simulink model "model2"  (R2022b)
settings: Solver=VariableStepAuto  StartTime=0.0  StopTime=0.5  RelTol=1e-3
libraries: simulink x1
settings Model: Creator=NINGMEI  LastModifiedBy=NINGMEI

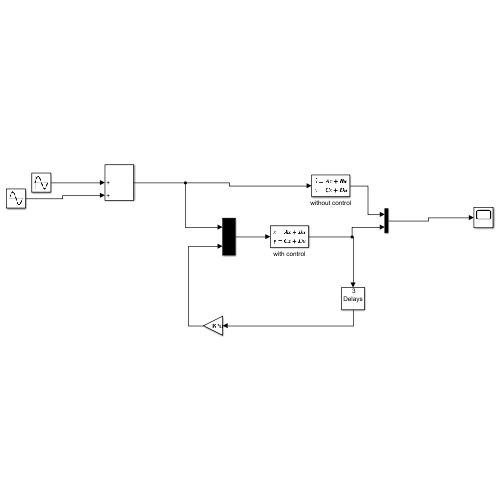
[thumbnail: Simulink's stored preview of the top-level diagram]
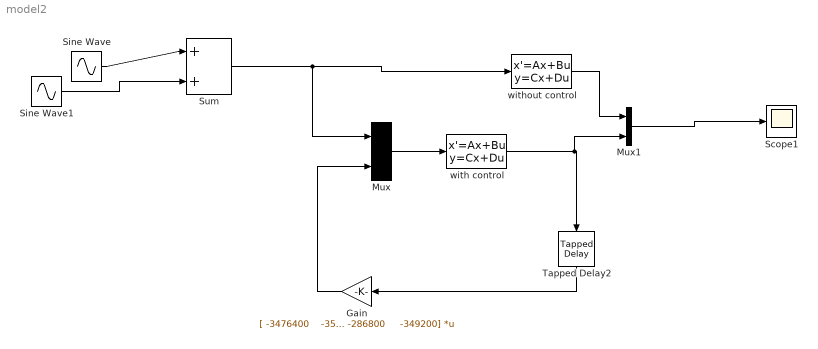
== system model2 ==
  Gain : Gain  Gain=|  Multiplication=Matrix(K*u)
      | [ -3476400    -3542000    -1883600     -702000
      |     -1159600    -1084400     -286800     -349200]
  Mux : Mux  Inputs=2
  Mux1 : Mux  Inputs=2
  Scope1 : Scope
  Sine Wave : Sin  Amplitude=1/2  Frequency=2*pi*106  SampleTime=0
  Sine Wave1 : Sin  Amplitude=1/2  Frequency=2*pi*76  SampleTime=0
  Sum : Sum  Inputs=|++
  Tapped Delay2 : simulink/Discrete/Tapped Delay  vinit=0.0  samptime=0.001  NumDelays=3  DelayOrder=Newest  includeCurrent=on
  with control : StateSpace  A=[0,1,0,0,0,0,0,0,0,0,0,0,0,0,0,0,0,0,0,0;-218756.663497404,-75.3943158453190,0,0,0,0,0,0,0,0,0,0,0,0,0,0,0,0,0,0;0,0,0,1,0,0,0,0,0,0,0,0,0,0,0,0,0,0,0,0;0,0,-425015.189785222,-121.227999776810,0,0,0,0,0,0,0,0,0,0,0,0,0,0,0,0;0,0,0,0,0,1,0,0,0,0,0,0,0,0,0,0,0,0,0,0;0,0,0,0,-1543652.61251911,-179.366262314666,0,0,0,0,0,0,0,0,0,0,0,0,0,0;0,0,0,0,0,0,0,1,0,0,0,0,0,0,0,0,0,0,0,0;0,0,0,0,0,0,-2081588.63244024,-143.313684770308,0,0,0,0,0,0,0,0,0,0,0,0;0,0,0,0,0,0,0,0,0,1,0,0,0,0,0,0,0,0,0,0;0,0,0,0,0,0,0,0,-2130030.47659911,-287.910764362321,0,0,0,0,0,0,0,0,0,0;0,0,0,0,0,0,0,0,0,0,0,1,0,0,0,0,0,0,0,0;0,0,0,0,0,0,0,0,0,0,-5305960.14059000,-288.771385034875,0,0,0,0,0,0,0,0;0,0,0,0,0,0,0,0,0,0,0,0,0,1,0,0,0,0,0,0;0,0,0,0,0,0,0,0,0,0,0,0,-5390944.25230139,-264.646348871112,0,0,0,0,0,0;0,0,0,0,0,0,0,0,0,0,0,0,0,0,0,1,0,0,0,0;0,0,0,0,0,0,0,0,0,0,0,0,0,0,-6091540.06991477,-379.473957868670,0,0,0,0;0,0,0,0,0,0,0,0,0,0,0,0,0,0,0,0,0,1,0,0;0,0,0,0,0,0,0,0,0,0,0,0,0,0,0,0,-9815859.08825058,-155.529954281920,0,0;0,0,0,0,0,0,0,0,0,0,0,0,0,0,0,0,0,0,0,1;0,0,0,0,0,0,0,0,0,0,0,0,0,0,0,0,0,0,-11663878.9371333,-288.313555742022]  B=|  C="[16.0376601050147\t0.425434196872911\t-35.4185444812321\t-0.584329437860915\t2.27495049096470e-10\t7.07661855623417e-13\t41.8170016588276\t0.583573044344012\t2.55088376318462e-10\t8.59942503205762e-13\t-1.72531236384178e-08\t1.11780139528277e-11\t-66.5566171517801\t-0.502985342028614\t-59.6684503519825\t-0.511944736456433\t-46.6516329782968\t-0.599905441928972\t71.1035666921190\t0.493237763380162]"  D=zeros(1,3)  InitialCondition=0
      | [-0.00130142918674408	1.30358515621439e-08	1.30358515745248e-08
      | -8.05097234388870	0.000161986493696331	0.000161986493698015
      | 0.00174521761973298	-2.26152627580204e-08	2.26152627898945e-08
      | 9.47255980317982	-0.000238132799911334	0.000238132799917303
      | -4.68558949874813e-14	-5.17251016726256e-18	2.78410120575176e-18
      | -6.36926525728054e-11	-6.97026713212352e-15	8.33102894791208e-15
      | -0.000688617320963496	4.00416374839661e-09	4.00416377115030e-09
      | -1.50303151591078	0.000194961141440238	0.000194961141449204
      | -3.27947145132250e-14	-1.36102631975034e-17	-1.45883041572654e-17
      | -2.13125349021250e-12	1.99965490207049e-15	-2.07329393701453e-14
      | 6.29305646918913e-14	5.10828688252961e-18	6.96617258686553e-18
      | 3.63273766667846e-11	-1.69282404711518e-15	3.17691424161274e-17
      | -0.000525656982902977	2.01866444434949e-08	2.01866444552086e-08
      | 6.86160066811968	-0.000115627228664429	-0.000115627228655436
      | -6.11888532734705e-05	-3.64677239026098e-09	3.64677231514311e-09
      | 7.71315083473833	-0.000208133722521158	0.000208133722428171
      | -0.000285899607555637	2.60751778707382e-08	-2.60751778004454e-08
      | -6.82543136934396	-0.000305159842494010	0.000305159842438341
      | -0.000209578204541874	1.56163736681111e-08	1.56163736543140e-08
      | -0.188064987868392	0.000383963826542559	0.000383963826539278]
  without control : StateSpace  A=[0,1,0,0,0,0,0,0,0,0,0,0,0,0,0,0,0,0,0,0;-218756.663497404,-75.3943158453190,0,0,0,0,0,0,0,0,0,0,0,0,0,0,0,0,0,0;0,0,0,1,0,0,0,0,0,0,0,0,0,0,0,0,0,0,0,0;0,0,-425015.189785222,-121.227999776810,0,0,0,0,0,0,0,0,0,0,0,0,0,0,0,0;0,0,0,0,0,1,0,0,0,0,0,0,0,0,0,0,0,0,0,0;0,0,0,0,-1543652.61251911,-179.366262314666,0,0,0,0,0,0,0,0,0,0,0,0,0,0;0,0,0,0,0,0,0,1,0,0,0,0,0,0,0,0,0,0,0,0;0,0,0,0,0,0,-2081588.63244024,-143.313684770308,0,0,0,0,0,0,0,0,0,0,0,0;0,0,0,0,0,0,0,0,0,1,0,0,0,0,0,0,0,0,0,0;0,0,0,0,0,0,0,0,-2130030.47659911,-287.910764362321,0,0,0,0,0,0,0,0,0,0;0,0,0,0,0,0,0,0,0,0,0,1,0,0,0,0,0,0,0,0;0,0,0,0,0,0,0,0,0,0,-5305960.14059000,-288.771385034875,0,0,0,0,0,0,0,0;0,0,0,0,0,0,0,0,0,0,0,0,0,1,0,0,0,0,0,0;0,0,0,0,0,0,0,0,0,0,0,0,-5390944.25230139,-264.646348871112,0,0,0,0,0,0;0,0,0,0,0,0,0,0,0,0,0,0,0,0,0,1,0,0,0,0;0,0,0,0,0,0,0,0,0,0,0,0,0,0,-6091540.06991477,-379.473957868670,0,0,0,0;0,0,0,0,0,0,0,0,0,0,0,0,0,0,0,0,0,1,0,0;0,0,0,0,0,0,0,0,0,0,0,0,0,0,0,0,-9815859.08825058,-155.529954281920,0,0;0,0,0,0,0,0,0,0,0,0,0,0,0,0,0,0,0,0,0,1;0,0,0,0,0,0,0,0,0,0,0,0,0,0,0,0,0,0,-11663878.9371333,-288.313555742022]  B=|  C="[16.0376601050147\t0.425434196872911\t-35.4185444812321\t-0.584329437860915\t2.27495049096470e-10\t7.07661855623417e-13\t41.8170016588276\t0.583573044344012\t2.55088376318462e-10\t8.59942503205762e-13\t-1.72531236384178e-08\t1.11780139528277e-11\t-66.5566171517801\t-0.502985342028614\t-59.6684503519825\t-0.511944736456433\t-46.6516329782968\t-0.599905441928972\t71.1035666921190\t0.493237763380162]"  D=0  InitialCondition=0
      | [-0.00130142918674408
      | -8.05097234388870
      | 0.00174521761973298
      | 9.47255980317982
      | -4.68558949874813e-14
      | -6.36926525728054e-11
      | -0.000688617320963496
      | -1.50303151591078
      | -3.27947145132250e-14
      | -2.13125349021250e-12
      | 6.29305646918913e-14
      | 3.63273766667846e-11
      | -0.000525656982902977
      | 6.86160066811968
      | -6.11888532734705e-05
      | 7.71315083473833
      | -0.000285899607555637
      | -6.82543136934396
      | -0.000209578204541874
      | -0.188064987868392]
  wires:
  Sine Wave/1 -> Sum/1
  Sine Wave1/1 -> Sum/2
  Sum/1 -> Mux/1, without control/1
  with control/1 -> Mux1/2, Tapped Delay2/1
  Tapped Delay2/1 -> Gain/1
  Mux/1 -> with control/1
  Gain/1 -> Mux/2
  without control/1 -> Mux1/1
  Mux1/1 -> Scope1/1
